simulink model "cp_sim_2"  (R2025b)
settings: Solver=ode45  StartTime=0.0  StopTime=10.0  MaxStep=1e-1  RelTol=1e-12  AbsTol=1e-12
settings Model: Creator=white  LastModifiedBy=white

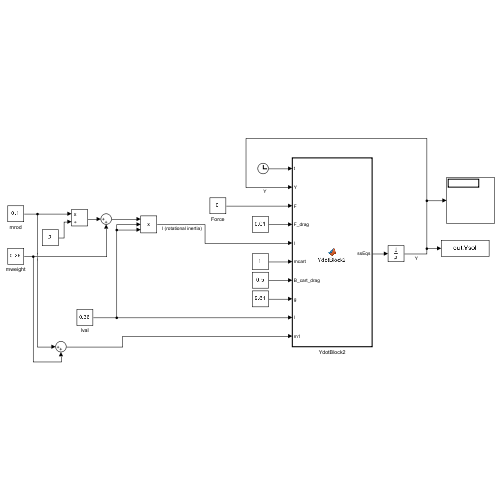
[thumbnail: Simulink's stored preview of the top-level diagram]
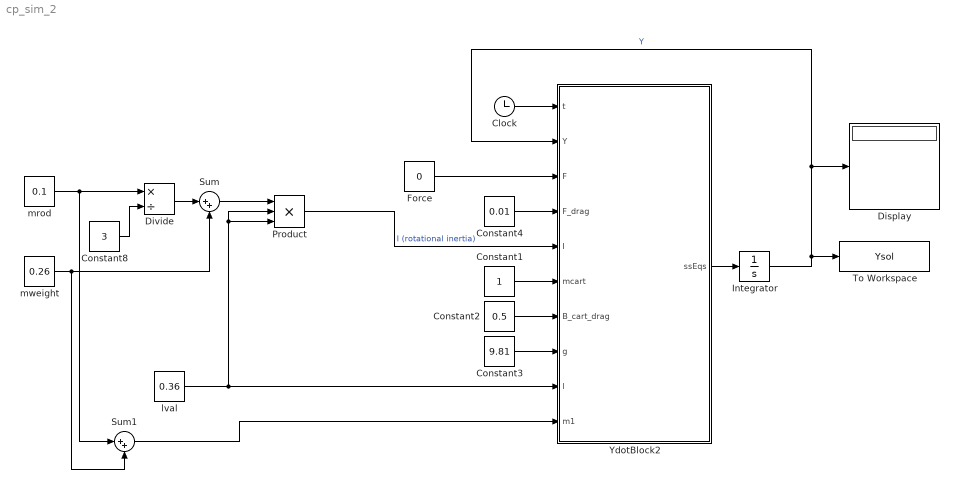
== system cp_sim_2 ==
  Clock : Clock
  Constant1 : Constant
  Constant2 : Constant  Value=0.5
  Constant3 : Constant  Value=9.81
  Constant4 : Constant  Value=0.01
  Constant8 : Constant  Value=3
  Display : Display
  Divide : Product  Inputs=*/
  Force : Constant  Value=0
  Integrator : Integrator
  Product : Product  Inputs=3
  Sum : Sum  Inputs=|++
  Sum1 : Sum  Inputs=|++
  To Workspace : ToWorkspace  VariableName=Ysol  SaveFormat=Structure With Time  SampleTime=-1
  YdotBlock2 : MATLAB Function  TreatAsAtomicUnit=on
  lval : Constant  Value=0.36
  mrod : Constant  Value=0.1
  mweight : Constant  Value=0.26
  wires:
  Integrator/1 -> Display/1, YdotBlock2/2(Y), To Workspace/1  "Y"
  Force/1 -> YdotBlock2/3(F)
  Constant4/1 -> YdotBlock2/4(F_drag)
  Sum1/1 -> YdotBlock2/10(m1)
  lval/1 -> YdotBlock2/9(l), Product/2, Product/3
  Constant3/1 -> YdotBlock2/8(g)
  Constant2/1 -> YdotBlock2/7(B_cart_drag)
  Constant1/1 -> YdotBlock2/6(mcart)
  Clock/1 -> YdotBlock2/1(t)
  YdotBlock2/1(ssEqs) -> Integrator/1
  Constant8/1 -> Divide/2
  mrod/1 -> Sum1/1, Divide/1
  Divide/1 -> Sum/1
  mweight/1 -> Sum1/2, Sum/2
  Sum/1 -> Product/1
  Product/1 -> YdotBlock2/5(I)  "I (rotational inertia)"

== matlab function cp_sim_2/YdotBlock2 ==
  data: t input; ssEqs output; Y input; F input; F_drag input; I input; mcart input; B_cart_drag input; g input; l input; m1 input
function ssEqs = YdotBlock2(t,Y,F,F_drag,I,mcart,B_cart_drag,g,l,m1)
%#codegen

ssEqs = zeros(4, 1);

% coder.extrinsic('disp', 'size');
% disp(size(ssEqs));
% 
% if numel(Y) < 4
%     error('Input Y has less than 4 elements. Size: %s', mat2str(size(Y)));
% end

%    This function was generated by the Symbolic Math Toolbox version 25.2.
%    08-Oct-2025 16:02:27

% t = complex(t);  % if required to enforce complex operations
% Y = complex(Y);  % if required to enforce complex operations
% F = complex(F);  % if required to enforce complex operations
% F_drag = complex(F_drag);  % if required to enforce complex operations
% I = complex(I);  % if required to enforce complex operations
% mcart = complex(mcart);  % if required to enforce complex operations
% B_cart_drag = complex(B_cart_drag);  % if required to enforce complex operations
% g = complex(g);  % if required to enforce complex operations
% l = complex(l);  % if required to enforce complex operations
% m1 = complex(m1);  % if required to enforce complex operations
t2 = I.*m1;
t3 = I.*mcart;
t4 = Y(1);
t5 = Y(2);
t6 = Y(4);
t7 = l.^2;
t8 = m1.^2;
t9 = cos(t4);
t10 = sin(t4);
t11 = t5.^2;
t12 = m1.*mcart.*t7;
t14 = t7.*t8;
t13 = t9.^2;
t15 = t13.*t14;
t16 = -t15;
t17 = t2+t3+t12+t14+t16;
t18 = 1.0./t17;
ssEqs = [t5;l.*t18.*(F.*m1.*t9+F_drag.*mcart.*t9+g.*t8.*t10+g.*m1.*mcart.*t10-B_cart_drag.*m1.*t6.*t9-l.*t8.*t9.*t10.*t11);t6;-t18.*(-F.*I+F_drag.*I+B_cart_drag.*I.*t6-F.*m1.*t7+F_drag.*m1.*t7-g.*t9.*t10.*t14+l.*t2.*t10.*t11+l.^3.*t8.*t10.*t11+B_cart_drag.*m1.*t6.*t7-F_drag.*m1.*t7.*t13)];

end
